simulink model "CalcThrust_v1"  (R2017b)
settings: Solver=VariableStepAuto  StartTime=0.0  StopTime=10.0  RelTol=1e-3
values from neighbouring files (symbols this model uses):
  Fmax = 2500    [ThrustEstimation.m]
  m = 1    [AB1Auf2.m]    (also in AB4Auf2.m = [1248 57153]; AB5Auf1.m = 7974)
  mu = 3.2    [ThrustEstimation.m]
  P_0 = 101325    [ThrustEstimation.m]
  rho_0 = 1.225    [ThrustEstimation.m]
  s = omega * 1i    [ABAuf1.m]
libraries: aerolibconvert2 x2, aerolibatmos2 x1
settings Model: Creator=danyc  LastModifiedBy=danyc

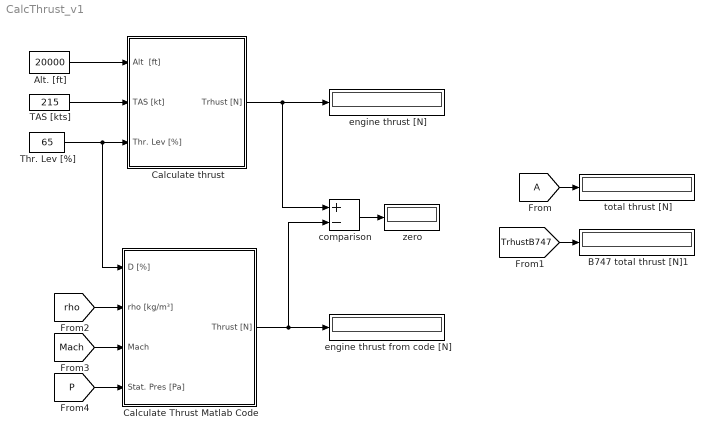
== system CalcThrust_v1 ==
  Alt. [ft] : Constant  Value=20000
  B747 total thrust [N]1 : Display
  Calculate Thrust Matlab Code : Subsystem
  Calculate thrust : Subsystem
  TAS [kts] : Constant  Value=215
  Thr. Lev [%] : Constant  Value=65
  comparison : Sum  Inputs=+-
  engine thrust [N] : Display
  engine thrust from code [N] : Display
  total thrust [N] : Display
  zero : Display
  wires:
  Calculate thrust/1(Trhust [N]) -> comparison/1, engine thrust [N]/1
  [A] -> total thrust [N]/1
  [TrhustB747] -> B747 total thrust [N]1/1
  Alt. [ft]/1 -> Calculate thrust/1(Alt  [ft])
  TAS [kts]/1 -> Calculate thrust/2(TAS [kt])
  Thr. Lev [%]/1 -> Calculate thrust/3(Thr. Lev [%]), Calculate Thrust Matlab Code/1(D [%])
  [rho] -> Calculate Thrust Matlab Code/2(rho [kg/m³])
  [Mach] -> Calculate Thrust Matlab Code/3(Mach)
  [P] -> Calculate Thrust Matlab Code/4(Stat. Pres [Pa])
  Calculate Thrust Matlab Code/1(Thrust [N]) -> comparison/2, engine thrust from code [N]/1
  comparison/1 -> zero/1

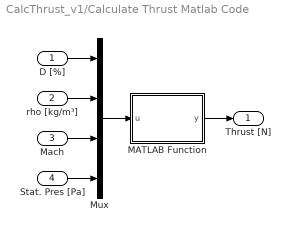
== system CalcThrust_v1/Calculate Thrust Matlab Code ==
  D [%] : Inport
  rho [kg/m³] : Inport  Port=2
  Mach : Inport  Port=3
  Stat. Pres [Pa] : Inport  Port=4
  MATLAB Function : MATLAB Function  TreatAsAtomicUnit=on
  Mux : Mux
  Thrust [N] : Outport
  wires:
  MATLAB Function/1(y) -> Thrust [N]/1
  Mux/1 -> MATLAB Function/1(u)
  D [%]/1 -> Mux/1
  Stat. Pres [Pa]/1 -> Mux/4
  rho [kg/m³]/1 -> Mux/2
  Mach/1 -> Mux/3

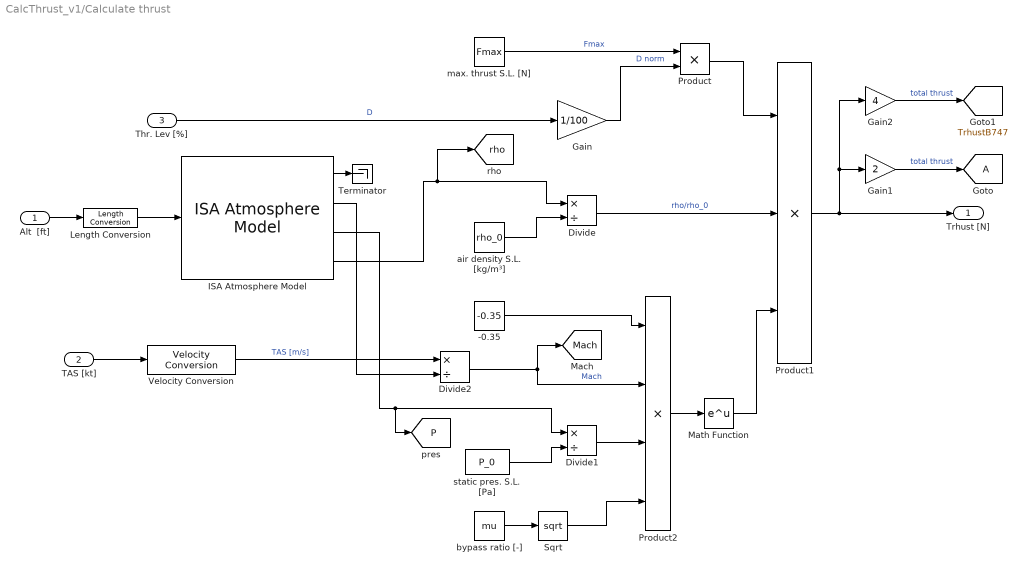
== system CalcThrust_v1/Calculate thrust ==
  Alt  [ft] : Inport
  TAS [kt] : Inport  Port=2
  Thr. Lev [%] : Inport  Port=3
  -0.35 : Constant  Value=-0.35
  Divide : Product  Inputs=*/
  Divide1 : Product  Inputs=*/
  Divide2 : Product  Inputs=*/
  Gain : Gain  Gain=1/100
  Gain1 : Gain  Gain=2
  Gain2 : Gain  Gain=4
  ISA Atmosphere Model : aerolibatmos2/ISA Atmosphere Model  custom=off  g=9.80665  gamma=1.4  R=287.0531  L=0.0065  h_trop=11000  h_strat=20000  rho0=1.225  P0=101325  T0=288.15  h0=0
      settings: SourceProductName=Aerospace Blockset
  Length Conversion : aerolibconvert2/Length Conversion  IU=ft  OU=m
  Math Function : Math  SaturateOnIntegerOverflow=on
  Product : Product
  Product1 : Product  Inputs=3
  Product2 : Product  Inputs=4
  Sqrt : Sqrt  SaturateOnIntegerOverflow=on
  Terminator : Terminator
  Velocity Conversion : aerolibconvert2/Velocity Conversion  IU=kts  OU=m/s
  air density S.L. [kg/m³] : Constant  Value=rho_0
  bypass ratio [-] : Constant  Value=mu
  max. thrust S.L. [N] : Constant  Value=Fmax
  static pres. S.L. [Pa] : Constant  Value=P_0
  Trhust [N] : Outport
  tag scope: A=global, Mach=global, P=global, TrhustB747=global, rho=global
  wires:
  Divide2/1 -> [Mach], Product2/2  "Mach"
  static pres. S.L. [Pa]/1 -> Divide1/2
  Divide1/1 -> Product2/3
  Math Function/1 -> Product1/3
  bypass ratio [-]/1 -> Sqrt/1
  Divide/1 -> Product1/2  "rho/rho_0"
  air density S.L. [kg/m³]/1 -> Divide/2
  -0.35/1 -> Product2/1
  ISA Atmosphere Model/4 -> [rho], Divide/1
  max. thrust S.L. [N]/1 -> Product/1  "Fmax"
  Thr. Lev [%]/1 -> Gain/1  "D"
  Product/1 -> Product1/1
  ISA Atmosphere Model/3 -> [P], Divide1/1
  Product2/1 -> Math Function/1
  Gain/1 -> Product/2  "D norm"
  Sqrt/1 -> Product2/4
  Product1/1 -> Gain2/1, Gain1/1, Trhust [N]/1
  Gain1/1 -> [A]  "total thrust"
  Gain2/1 -> [TrhustB747]  "total thrust"
  ISA Atmosphere Model/2 -> Divide2/2
  Velocity Conversion/1 -> Divide2/1  "TAS [m/s]"
  ISA Atmosphere Model/1 -> Terminator/1
  Alt  [ft]/1 -> Length Conversion/1
  Length Conversion/1 -> ISA Atmosphere Model/1
  TAS [kt]/1 -> Velocity Conversion/1

== matlab function CalcThrust_v1/Calculate Thrust Matlab Code/MATLAB Function ==
  data: u input; y output
function y = fcn(u)

%  Parameters
Fmax    = 2500;         % maximum engine thrust [N]
mu      = 3.2;       	% engine bypass ratio
rho_0   = 1.225;     	% air density at sea level [kg/m³]
P_0     = 101325;     	% static air pressure at sea level [Pa]

% Variables 
D       = u(1);         % throttle lever position [%]  
rho     = u(2);         % air density at flight level [kg/m³]
Ma      = u(3);         % Mach number
P       = u(4);         % static pressure at flight altitude [Pa]

% Code
% engine thrust [N]
F = Fmax * (D / 100) * (rho / rho_0) * exp(-0.35 * Ma * (P / P_0) * sqrt(mu));

y = F;
